simulink model "Interstellar21"  (R2020a)
settings: Solver=ode3  StartTime=0  StopTime=TFinal  FixedStep=Ts  RelTol=1e-3  EnableMultiTasking=on
undefined symbols (not defined in the file or in its folder): bbox_edge_distance_threshold, g, gray, max_num_blobs, Rec, rho, SDTV, sensorCalibrationData, Sensors, sigbuilder_block, States, strel, takeOffDuration
libraries: simulink x14, liblinearframe x1, libraries_plantLibrary x1, visionfilter x1, visionmorphops x1, visionanalysis x1, visionstatistics x1, visiontextngfix x1, visionconversions x1, sensorsLibrary x1
settings Model: Creator=The MathWorks, Inc.  LastModifiedBy=User
settings DataIOCC: LimitDataPoints=on  SaveFormat=Array  SaveOutput=off  SignalLogging=off  DSMLogging=off  SaveTime=off  ReturnWorkspaceOutputs=off
settings OptimizationCC: BlockReduction=off  BufferReuse=off  LifeSpan=inf
settings DebuggingCC: AlgebraicLoopMsg=none  ParameterPrecisionLossMsg=none  UnconnectedInputMsg=none  UnconnectedOutputMsg=none  UnconnectedLineMsg=none  AllowSymbolicDim=off  SFUnexpectedBacktrackingDiag=warning  SFNoUnconditionalDefaultTransitionDiag=warning  SFExecutionAtInitializationDiag=none  ArithmeticOperatorsInVariantConditions=warning
settings HardwareCC: ProdBitPerPointer=32  ProdBitPerSizeT=32  ProdBitPerPtrDiffT=32  ProdLargestAtomicFloat=None  ProdIntDivRoundTo=Undefined  ProdEndianess=Unspecified  ProdWordSize=32  ProdHWDeviceType=32-bit Generic
settings ModelReferenceCC: PropagateSignalLabelsOutOfModel=off
settings SFSimCC: SimUseLocalCustomCode=off  CustomCodeUndefinedFunction=UseInterfaceOnly
settings RTWCC: RTWUseLocalCustomCode=off
settings CodeAppCC: StateflowObjectComments=on
settings GRTTargetCC: TargetLangStandard=C89/C90 (ANSI)
settings ConfigComp: CovMetricSettings=dw  CovHtmlReporting=on  CovSaveCumulativeToWorkspaceVar=on  CovSaveSingleToWorkspaceVar=on  CovExternalEMLEnable=off  CovSFcnEnable=off

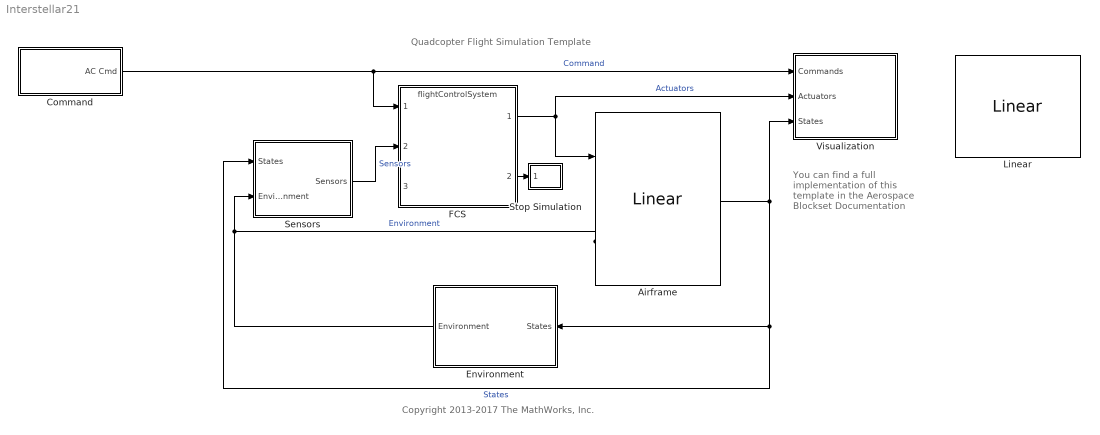
== system Interstellar21 ==
  note: You can find a full implementation of this template in the
      | Aerospace Blockset Documentation
  note: Quadcopter Flight Simulation Template
  note: Copyright 2013-2017 The MathWorks, Inc.
  Airframe : liblinearframe/Linear  SystemSampleTime=-1  Latency=0  AutoFrameSizeCalculation=off
  Command : Subsystem  VariantControl=VSS_COMMAND_SIGBLDR
  Environment : Subsystem  TreatAsAtomicUnit=on  VariantControl=VSS_ENVIRONMENT_CST
  FCS : ModelReference  ModelNameDialog=flightControlSystem.slx  SimulationMode=Normal  ModelReferenceVersion=1.137
  Linear : libraries_plantLibrary/Linear  SystemSampleTime=-1  Latency=0  AutoFrameSizeCalculation=off
  Sensors : Subsystem  TreatAsAtomicUnit=on  VariantControl=VSS_SENSORS_FEEDTHROUGH
  Stop Simulation : Subsystem
  Visualization : Subsystem  VariantControl=VSS_VISUALIZATION_SCOPES
  wires:
  Command/1(AC Cmd) -> Visualization/1(Commands), FCS/1  "Command"
  Sensors/1(Sensors) -> FCS/2  "Sensors"
  FCS/1 -> Airframe/1, Visualization/2(Actuators)  "Actuators"
  Environment/1(Environment) -> Airframe/2, Sensors/2(Environment)  "Environment"
  Airframe/1 -> Visualization/3(States), Environment/1(States), Sensors/1(States)  "States"
  FCS/2 -> Stop Simulation/1(Flag)

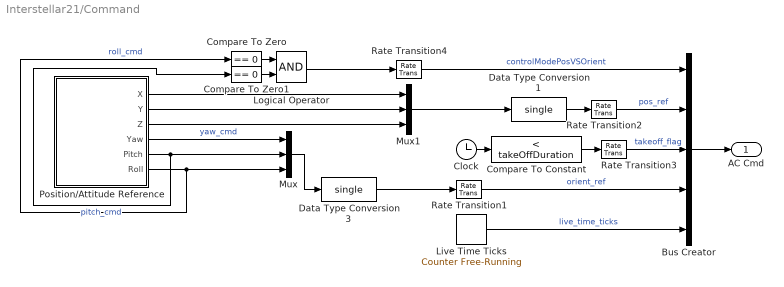
== system Interstellar21/Command ==
  Bus Creator : BusCreator  Inputs=5  OutDataTypeStr=Bus: CommandBus  NonVirtualBus=on
  Clock : Clock
  Compare To Constant : simulink/Logic and Bit Operations/Compare To Constant  relop=<  const=takeOffDuration  OutDataTypeStr=boolean
  Compare To Zero : simulink/Logic and Bit Operations/Compare To Zero  relop===  OutDataTypeStr=boolean
  Compare To Zero1 : simulink/Logic and Bit Operations/Compare To Zero  relop===  OutDataTypeStr=boolean
  Data Type Conversion1 : DataTypeConversion  OutDataTypeStr=single
  Data Type Conversion3 : DataTypeConversion  OutDataTypeStr=single
  Live Time Ticks : simulink/Sources/Counter Free-Running  NumBits=32  tsamp=Ts
  Logical Operator : Logic  AllPortsSameDT=off  OutDataTypeStr=boolean
  Mux : Mux  Inputs=3
  Mux1 : Mux  Inputs=3
  Position/Attitude Reference : Subsystem  Tag=STV Subsys  LoadFcn=sigbuilder_block('load');  StartFcn=sigbuilder_block('start');  StopFcn=sigbuilder_block('stop');  ClipboardFcn=sigbuilder_block('clipboard');  mask(Sigbuilder block){tuvar=[0:10]}
      mask help: Simulink:masks:SigbuilderBlock_MD
      mask init:
      | if ~strcmp(get_param(bdroot(gcbh),'SimulationStatus'),'stopped') tuvar = sigbuilder_block('maskInit'); end
      settings: CopyFcn=sigbuilder_block('copy');  DeleteFcn=sigbuilder_block('delete');  ModelCloseFcn=sigbuilder_block('modelClose');  PreSaveFcn=sigbuilder_block('preSave');  PauseFcn=sigbuilder_block('pause');  ContinueFcn=sigbuilder_block('continue');  NameChangeFcn=sigbuilder_block('namechange');  OpenFcn=sigbuilder_block('open',[246 211.5 555 408.75 ]);  CloseFcn=sigbuilder_block('close');
      mask Display: plot(0, 0, 100, 100,[2, 2, 32, 32, 2], [68, 8, 8, 68, 68],[32, 2], [38, 38], [32, 19, 2],[53, 60, 44], [32, 17, 17, 2],[16, 16, 31, 31]);txt = getActiveGroup(gcbh);text(2, 100, txt,'verticalAlignment', 'top');
  Rate Transition{1..4} (4 alike) : RateTransition  OutPortSampleTime=Ts
  AC Cmd : Outport  OutDataTypeStr=Bus: CommandBus  VectorParamsAs1DForOutWhenUnconnected=off
  wires:
  Bus Creator/1 -> AC Cmd/1
  Position/Attitude Reference/6(Roll) -> Compare To Zero/1, Mux/3  "roll_cmd"
  Position/Attitude Reference/5(Pitch) -> Mux/2, Compare To Zero1/1  "pitch_cmd"
  Position/Attitude Reference/4(Yaw) -> Mux/1  "yaw_cmd"
  Mux/1 -> Data Type Conversion3/1
  Data Type Conversion3/1 -> Rate Transition1/1
  Rate Transition1/1 -> Bus Creator/4  "orient_ref"
  Compare To Zero/1 -> Logical Operator/1
  Compare To Zero1/1 -> Logical Operator/2
  Logical Operator/1 -> Rate Transition4/1
  Rate Transition4/1 -> Bus Creator/1  "controlModePosVSOrient"
  Position/Attitude Reference/1(X) -> Mux1/1
  Position/Attitude Reference/2(Y) -> Mux1/2
  Position/Attitude Reference/3(Z) -> Mux1/3
  Mux1/1 -> Data Type Conversion1/1
  Data Type Conversion1/1 -> Rate Transition2/1
  Rate Transition2/1 -> Bus Creator/2  "pos_ref"
  Clock/1 -> Compare To Constant/1
  Compare To Constant/1 -> Rate Transition3/1
  Rate Transition3/1 -> Bus Creator/3  "takeoff_flag"
  Live Time Ticks/1 -> Bus Creator/5  "live_time_ticks"

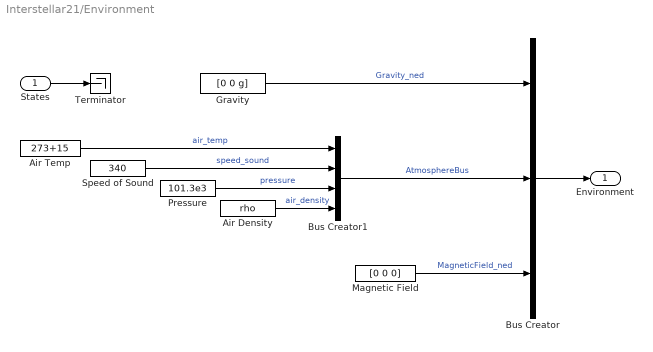
== system Interstellar21/Environment ==
  States : Inport  OutDataTypeStr=Bus: StatesBus
  Air Density : Constant  Value=rho
  Air Temp : Constant  Value=273+15
  Bus Creator : BusCreator  Inputs=3  OutDataTypeStr=Bus: EnvironmentBus  NonVirtualBus=on
  Bus Creator1 : BusCreator  Inputs=4  OutDataTypeStr=Bus: AtmosphereBus  NonVirtualBus=on
  Gravity : Constant  Value=[0 0 g]
  Magnetic Field : Constant  Value=[0 0 0]
  Pressure : Constant  Value=101.3e3
  Speed of Sound : Constant  Value=340
  Terminator : Terminator
  Environment : Outport  VectorParamsAs1DForOutWhenUnconnected=off
  wires:
  States/1 -> Terminator/1
  Gravity/1 -> Bus Creator/1  "Gravity_ned"
  Bus Creator/1 -> Environment/1
  Air Temp/1 -> Bus Creator1/1  "air_temp"
  Speed of Sound/1 -> Bus Creator1/2  "speed_sound"
  Pressure/1 -> Bus Creator1/3  "pressure"
  Air Density/1 -> Bus Creator1/4  "air_density"
  Bus Creator1/1 -> Bus Creator/2  "AtmosphereBus"
  Magnetic Field/1 -> Bus Creator/3  "MagneticField_ned"

== system Interstellar21/Sensors ==
  States : Inport  OutDataTypeStr=Bus: StatesBus
  Environment : Inport  Port=2  OutDataTypeStr=Bus: EnvironmentBus
  Bus Creator1 : BusCreator  Inputs=3  OutDataTypeStr=Bus: SensorsBus  NonVirtualBus=on
  Bus Creator2 : BusCreator  Inputs=3  OutDataTypeStr=Bus: extraSensorData_t  NonVirtualBus=on
  Constant1 : Constant  Value=sensorCalibrationData  OutDataTypeStr=single
  Memory : Memory  InitialCondition=States  InheritSampleTime=on
  Sensor System : Subsystem
  _DUMMY_FLAG_usePosVIS : Constant  Value=Sensors.dummy.usePosVISFlag  OutDataTypeStr=single
  _DUMMY_posVIS : Constant  Value=Sensors.dummy.posVISNoVisionAvail  OutDataTypeStr=single
  Sensors : Outport  OutDataTypeStr=Bus: SensorsBus  VectorParamsAs1DForOutWhenUnconnected=off
  wires:
  Constant1/1 -> Bus Creator1/3  "SensorCalibration"
  Memory/1 -> Sensor System/1(States)
  Sensor System/2(sensordata_data) -> Bus Creator1/2  "HALSensor"
  States/1 -> Memory/1
  Environment/1 -> Sensor System/2(Environment)
  Bus Creator1/1 -> Sensors/1
  _DUMMY_FLAG_usePosVIS/1 -> Bus Creator2/3  "usePosVIS_flag"
  Sensor System/1(opticalFlow_data) -> Bus Creator2/1  "opticalFlow_data"
  _DUMMY_posVIS/1 -> Bus Creator2/2  "posVIS_data"
  Bus Creator2/1 -> Bus Creator1/1  "VisionSensors"

== system Interstellar21/Stop Simulation ==
  Flag : Inport
  Assertion : Assertion
  Compare To Zero : simulink/Logic and Bit Operations/Compare To Zero  relop=>  OutDataTypeStr=boolean
  Logical Operator : Logic  Operator=NOT  AllPortsSameDT=off  OutDataTypeStr=boolean
  wires:
  Flag/1 -> Compare To Zero/1
  Compare To Zero/1 -> Logical Operator/1
  Logical Operator/1 -> Assertion/1

== system Interstellar21/Visualization ==
  Commands : Inport  OutDataTypeStr=Bus: CommandBus
  Actuators : Inport  Port=2
  States : Inport  Port=3  OutDataTypeStr=Bus: StatesBus
  Bus Creator : BusCreator  Inputs=2
  Bus Selector : BusSelector  OutputSignals=States.V_body,States.Euler,States.X_ned
  Euler : Scope
  Motors : Scope
  V_body : Scope
  X_ned : Scope
  wires:
  Commands/1 -> Bus Creator/1  "Commands"
  States/1 -> Bus Creator/2  "States"
  Bus Creator/1 -> Bus Selector/1
  Bus Selector/1 -> V_body/1  "<V_body>"
  Bus Selector/2 -> Euler/1  "<Euler>"
  Bus Selector/3 -> X_ned/1  "<X_ned>"
  Actuators/1 -> Motors/1

== system Interstellar21/Command/Position//Attitude Reference ==
  Demux : Demux  Tag=STV Demux  Outputs=6
      settings: DisplayOption=none
  FromWs : FromWorkspace  Tag=STV FromWs  VariableName=tuvar
      SigBuilderData=|
      | common.afterFinalStr = 'Extrapolate'
      | common.sampleTime = 0
      | dataSet.timeRange = [0 100]
      | dataSet.name = 'Group 1'
      | sbobj.Groups.Name = 'Group 1'
      | sbobj.Groups.Signals(1).Name = 'X'
      | sbobj.Groups.Signals(1).XData = [0 100]
      | sbobj.Groups.Signals(1).YData = [0 0]
      | sbobj.Groups.Signals(2).Name = 'Y'
      | sbobj.Groups.Signals(2).XData = [0 100]
      | sbobj.Groups.Signals(2).YData = [0 0]
      | sbobj.Groups.Signals(3).Name = 'Z'
      | sbobj.Groups.Signals(3).XData = [0 1 1 100]
      | sbobj.Groups.Signals(3).YData = [0 0 -1.5 -1.5]
      | sbobj.Groups.Signals(4).Name = 'Yaw'
      | sbobj.Groups.Signals(4).XData = [0 5.5 8 100]
      | sbobj.Groups.Signals(4).YData = [0 0 0 0]
      | sbobj.Groups.Signals(5).Name = 'Pitch'
      | sbobj.Groups.Signals(5).XData = [0 3 4 100]
      | sbobj.Groups.Signals(5).YData = [0 0 0 0]
      | sbobj.Groups.Signals(6).Name = 'Roll'
      | sbobj.Groups.Signals(6).XData = [0 100]
      | sbobj.Groups.Signals(6).YData = [0 0]
      | sbobj.Groups.TimeRange = [0 100]
  X : Outport  Tag=STV Outport  VectorParamsAs1DForOutWhenUnconnected=off
  Y : Outport  Tag=STV Outport  Port=2  VectorParamsAs1DForOutWhenUnconnected=off
  Z : Outport  Tag=STV Outport  Port=3  VectorParamsAs1DForOutWhenUnconnected=off
  Yaw : Outport  Tag=STV Outport  Port=4  VectorParamsAs1DForOutWhenUnconnected=off
  Pitch : Outport  Tag=STV Outport  Port=5  VectorParamsAs1DForOutWhenUnconnected=off
  Roll : Outport  Tag=STV Outport  Port=6  VectorParamsAs1DForOutWhenUnconnected=off
  wires:
  FromWs/1 -> Demux/1
  Demux/1 -> X/1
  Demux/2 -> Y/1
  Demux/3 -> Z/1
  Demux/4 -> Yaw/1
  Demux/5 -> Pitch/1
  Demux/6 -> Roll/1

== system Interstellar21/Sensors/Sensor System ==
  States : Inport
  Environment : Inport  Port=2
  Camera : Subsystem  AncestorBlock=sensorsLibrary/Camera
  IMU_Pressure : Subsystem
  Rate Transition1 : RateTransition  OutPortSampleTime=Ts
  Rate Transition2 : RateTransition  OutPortSampleTime=Ts
  opticalFlow_data : Outport  VectorParamsAs1DForOutWhenUnconnected=off
  sensordata_data : Outport  Port=2  OutDataTypeStr=Bus: HAL_acquisition_t  VectorParamsAs1DForOutWhenUnconnected=off
  wires:
  Environment/1 -> IMU_Pressure/2(Environment)
  Camera/1(opticalFlow_datout) -> Rate Transition1/1
  IMU_Pressure/1(sensordata_datout) -> Rate Transition2/1
  Rate Transition1/1 -> opticalFlow_data/1
  Rate Transition2/1 -> sensordata_data/1
  States/1 -> Camera/1(states), IMU_Pressure/1(states_datin)

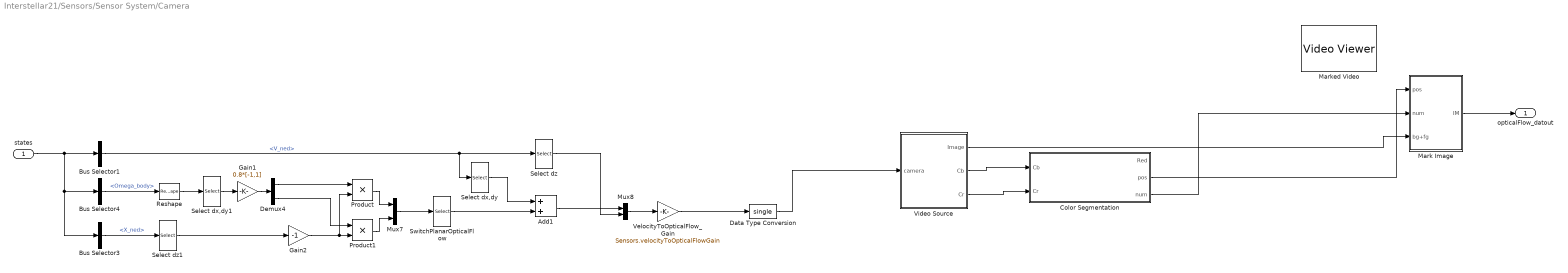
== system Interstellar21/Sensors/Sensor System/Camera ==
  states : Inport
  Add1 : Sum
  Bus Selector1 : BusSelector  OutputSignals=V_ned
  Bus Selector3 : BusSelector  OutputSignals=X_ned
  Bus Selector4 : BusSelector  OutputSignals=Omega_body
  Color Segmentation : Subsystem
  Data Type Conversion : DataTypeConversion  OutDataTypeStr=single
  Demux4 : Demux  Outputs=2
  Gain1 : Gain  Gain=0.8*[-1,1]
  Gain2 : Gain  Gain=-1
  Mark Image : Subsystem
  Marked Video : VideoViewer  colormapValue=gray(256)  FigPos=[410 344 166 142]  trueSizedOnce=on
  Mux7 : Mux  Inputs=2
  Mux8 : Mux  Inputs=2
  Product : Product
  Product1 : Product
  Reshape : Reshape
  Select dx,dy : Selector  InputPortWidth=3  IndexOptions=Index vector (dialog)  Indices=[1 2]  OutputSizes=1
  Select dx,dy1 : Selector  InputPortWidth=3  IndexOptions=Index vector (dialog)  Indices=[1 2]  OutputSizes=1
  Select dz : Selector  InputPortWidth=3  IndexOptions=Index vector (dialog)  Indices=3  OutputSizes=1
  Select dz1 : Selector  InputPortWidth=3  IndexOptions=Index vector (dialog)  Indices=3  OutputSizes=1
  SwitchPlanarOpticalFlow : Selector  InputPortWidth=2  IndexOptions=Index vector (dialog)  Indices=[2 1]  OutputSizes=1
  VelocityToOpticalFlow_Gain : Gain  Gain=Sensors.velocityToOpticalFlowGain
  "Video Source " : Subsystem
  opticalFlow_datout : Outport  VectorParamsAs1DForOutWhenUnconnected=off
  wires:
  Data Type Conversion/1 -> "Video Source "/1("camera ")
  Reshape/1 -> Select dx,dy1/1
  Select dz1/1 -> Gain2/1
  VelocityToOpticalFlow_Gain/1 -> Data Type Conversion/1
  Mux8/1 -> VelocityToOpticalFlow_Gain/1
  Bus Selector4/1 -> Reshape/1  "<Omega_body>"
  Bus Selector3/1 -> Select dz1/1  "<X_ned>"
  Select dz/1 -> Mux8/2
  Add1/1 -> Mux8/1
  SwitchPlanarOpticalFlow/1 -> Add1/2
  Select dx,dy/1 -> Add1/1
  Gain2/1 -> Product1/2, Product/2
  Select dx,dy1/1 -> Gain1/1
  Mux7/1 -> SwitchPlanarOpticalFlow/1
  Product1/1 -> Mux7/2
  Product/1 -> Mux7/1
  Demux4/2 -> Product1/1
  Gain1/1 -> Demux4/1
  Demux4/1 -> Product/1
  Bus Selector1/1 -> Select dz/1, Select dx,dy/1  "<V_ned>"
  states/1 -> Bus Selector1/1, Bus Selector4/1, Bus Selector3/1
  "Video Source "/1(Image) -> Mark Image/3(bg+fg)
  Color Segmentation/2(pos) -> Mark Image/1(pos)
  "Video Source "/3(Cr) -> Color Segmentation/2(Cr)
  Color Segmentation/3(num) -> Mark Image/2(num)
  "Video Source "/2(Cb) -> Color Segmentation/1(Cb)
  Mark Image/1(IM) -> opticalFlow_datout/1

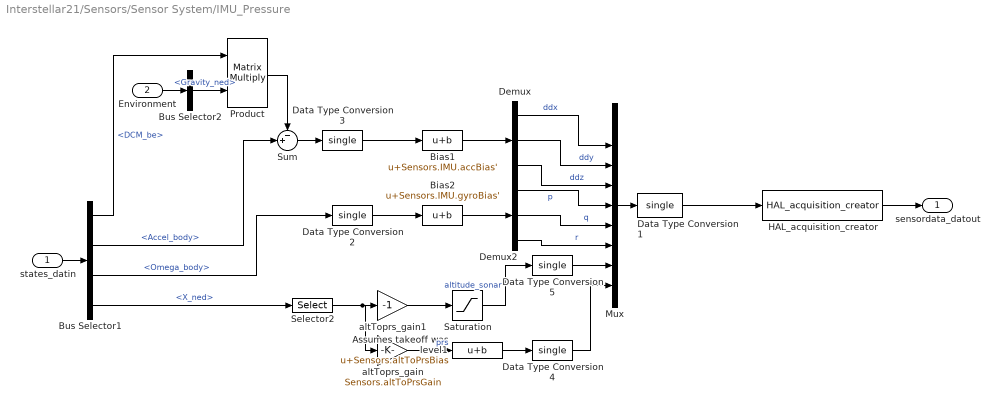
== system Interstellar21/Sensors/Sensor System/IMU_Pressure ==
  states_datin : Inport  OutDataTypeStr=Bus: StatesBus
  Environment : Inport  Port=2
  Assumes takeoff was level1 : Bias  Bias=Sensors.altToPrsBias
  Bias1 : Bias  Bias=Sensors.IMU.accBias'
  Bias2 : Bias  Bias=Sensors.IMU.gyroBias'
  Bus Selector1 : BusSelector  OutputSignals=DCM_be,Accel_body,Omega_body,X_ned
  Bus Selector2 : BusSelector  OutputSignals=Gravity_ned
  Data Type Conversion{1..5} (5 alike) : DataTypeConversion  OutDataTypeStr=single
  Demux : Demux  Outputs=3
  Demux2 : Demux  Outputs=3
  HAL_acquisition_creator : sensorsLibrary/HAL_acquisition_creator  SystemSampleTime=-1  Latency=0  AutoFrameSizeCalculation=off
  Mux : Mux  Inputs=9
  Product : Product  Multiplication=Matrix(*)
  Saturation : Saturate  UpperLimit=inf  LowerLimit=Sensors.altSensorMin  OutDataTypeStr=single
  Selector2 : Selector  InputPortWidth=3  IndexOptions=Index vector (dialog)  Indices=[3]  OutputSizes=1
  Sum : Sum  Inputs=-+|
  altToprs_gain : Gain  Gain=Sensors.altToPrsGain  ParamDataTypeStr=single  OutDataTypeStr=single
  altToprs_gain1 : Gain  Gain=-1  ParamDataTypeStr=single  OutDataTypeStr=single
  sensordata_datout : Outport  OutDataTypeStr=Bus: HAL_acquisition_t  VectorParamsAs1DForOutWhenUnconnected=off
  wires:
  Bias2/1 -> Demux2/1
  Bias1/1 -> Demux/1
  Product/1 -> Sum/1
  Bus Selector1/2 -> Sum/2  "<Accel_body>"
  Sum/1 -> Data Type Conversion3/1
  Bus Selector1/1 -> Product/1  "<DCM_be>"
  Bus Selector2/1 -> Product/2  "<Gravity_ned>"
  altToprs_gain1/1 -> Saturation/1
  Data Type Conversion5/1 -> Mux/8
  Data Type Conversion4/1 -> Mux/9
  Data Type Conversion2/1 -> Bias2/1
  Data Type Conversion3/1 -> Bias1/1
  Assumes takeoff was level1/1 -> Data Type Conversion4/1
  Bus Selector1/4 -> Selector2/1  "<X_ned>"
  states_datin/1 -> Bus Selector1/1
  Environment/1 -> Bus Selector2/1
  Bus Selector1/3 -> Data Type Conversion2/1  "<Omega_body>"
  HAL_acquisition_creator/1 -> sensordata_datout/1
  Data Type Conversion1/1 -> HAL_acquisition_creator/1
  Mux/1 -> Data Type Conversion1/1
  altToprs_gain/1 -> Assumes takeoff was level1/1  "prs"
  Saturation/1 -> Data Type Conversion5/1  "altitude_sonar"
  Selector2/1 -> altToprs_gain1/1, altToprs_gain/1
  Demux/3 -> Mux/4  "ddz"
  Demux2/3 -> Mux/7  "r"
  Demux/2 -> Mux/3  "ddy"
  Demux/1 -> Mux/2  "ddx"
  Demux2/1 -> Mux/5  "p"
  Demux2/2 -> Mux/6  "q"

== system Interstellar21/Sensors/Sensor System/Camera/Color Segmentation ==
  Cb : Inport
  Cr : Inport  Port=2
  Color Classifier : Subsystem
  Filtering : Subsystem
  Region Filtering : Subsystem
  "Red " : Outport
  pos : Outport  Port=2
  num : Outport  Port=3
  wires:
  Color Classifier/1("Red ") -> Filtering/1(Red)
  Filtering/1("refined Red ") -> "Red "/1, Region Filtering/1(Red)
  Cb/1 -> Color Classifier/1(cb)
  Cr/1 -> Color Classifier/2(cr)
  Region Filtering/1(Regions) -> pos/1
  Region Filtering/2(Count) -> num/1

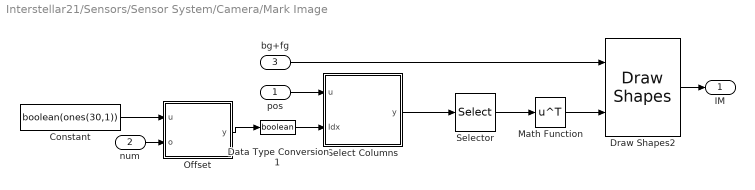
== system Interstellar21/Sensors/Sensor System/Camera/Mark Image ==
  pos : Inport
  num : Inport  Port=2
  bg+fg : Inport  Port=3
  Constant : Constant  Value=boolean(ones(30,1))
  Data Type Conversion1 : DataTypeConversion  OutDataTypeStr=boolean
  Draw Shapes2 : visiontextngfix/Draw Shapes  shape=Lines  fill=off  lineWidth=1  fillClrSource=Specify via dialog  display=User-specified value  intensity=200  color=[0 1 1]  opacity=0.6  viewport=Entire image  antialiasing=off  inType=Obsolete  imagePorts=One multidimensional signal  roundingMode=Floor  overflowMode=off  memoryMode=Specify word length  memoryWordLength=16  prodOutputMode=Binary point scaling  prodOutputWordLength=32  prodOutputFracLength=14  memoryFracLength=15
  Math Function : Math  Operator=transpose  SignedPower=on  SaturateOnIntegerOverflow=on
  Offset : MATLAB Function  TreatAsAtomicUnit=on
  Select Columns : MATLAB Function  TreatAsAtomicUnit=on
  Selector : Selector  NumberOfDimensions=2  InputPortWidth=3  IndexOptions=Index vector (dialog),Select all  Indices=[2 1 4 3],1  OutputSizes=1,1
  IM : Outport
  wires:
  Draw Shapes2/1 -> IM/1
  Data Type Conversion1/1 -> Select Columns/2(Idx)
  Constant/1 -> Offset/1(u)
  pos/1 -> Select Columns/1(u)
  num/1 -> Offset/2(o)
  bg+fg/1 -> Draw Shapes2/1
  Selector/1 -> Math Function/1
  Select Columns/1(y) -> Selector/1
  Math Function/1 -> Draw Shapes2/2
  Offset/1(y) -> Data Type Conversion1/1

== system Interstellar21/Sensors/Sensor System/Camera/Video Source  ==
  "camera " : Inport
  Color Space Conversion : visionconversions/Color Space  Conversion  conversion=Obsolete  conversionActive=R'G'B' to Y'CbCr  wp_str=D65  rec=Rec. 601 (SDTV)  sys=1125/60/2:1  imagePorts=One multidimensional signal
  Select Cb : Selector  NumberOfDimensions=3  InputPortWidth=3  IndexOptions=Select all,Select all,Index vector (dialog)  Indices=[1 3],1,2  OutputSizes=1,1,1
  Select Cr : Selector  NumberOfDimensions=3  InputPortWidth=3  IndexOptions=Select all,Select all,Index vector (dialog)  Indices=[1 3],1,3  OutputSizes=1,1,1
  Image : Outport
  Cb : Outport  Port=2
  Cr : Outport  Port=3
  wires:
  "camera "/1 -> Image/1, Color Space Conversion/1
  Color Space Conversion/1 -> Select Cb/1, Select Cr/1
  Select Cb/1 -> Cb/1
  Select Cr/1 -> Cr/1

== system Interstellar21/Sensors/Sensor System/Camera/Color Segmentation/Color Classifier ==
  cb : Inport
  cr : Inport  Port=2
  2-D FIR Filter : visionfilter/2-D FIR Filter  separable=off  filtSrc=Specify via dialog  filterMtrx=single(1/9*ones(3))  verticalFilter=[4 0]  horizontalFilter=[4 0]  outSize=Full  padType=Constant  padSrc=Specify via dialog  padVal=0  method=Convolution  firstCoeffSignedness=Signed  firstCoeffLastDataTypeStr=Inherit: Same word length as input  outputMode=Binary point scaling  outputWordLength=32  outputFracLength=12  outputSignedness=Auto  outputLastDataTypeStr=fixdt([],32,12)  accumLastDataTypeStr=Inherit: Same as product output  prodOutputMode=Binary point scaling  prodOutputWordLength=32  prodOutputFracLength=10  prodOutputLastDataTypeStr=fixdt([],32,10)  roundingMode=Floor  overflowMode=off  firstCoeffDataTypeStr=Inherit: Same word length as input  firstCoeffMin=[]  firstCoeffMax=[]  prodOutputDataTypeStr=fixdt([],32,10)  accumDataTypeStr=Inherit: Same as product output  outputDataTypeStr=fixdt([],32,12)  outputMin=[]  outputMax=[]
      settings: SourceProductBaseCode=VP
  Compare To Constant1 : simulink/Logic and Bit Operations/Compare To Constant  relop=<  const=2.5  OutDataTypeStr=boolean  ZeroCross=off
  "Mahalanobis Distance " : Subsystem
  "Red " : Outport
  wires:
  "Mahalanobis Distance "/1(Distance) -> 2-D FIR Filter/1
  cb/1 -> "Mahalanobis Distance "/1(Cb)
  cr/1 -> "Mahalanobis Distance "/2(Cr)
  Compare To Constant1/1 -> "Red "/1
  2-D FIR Filter/1 -> Compare To Constant1/1

== system Interstellar21/Sensors/Sensor System/Camera/Color Segmentation/Filtering ==
  Red : Inport
  Closing : visionmorphops/Closing  nhoodsrc=Specify via dialog  strel=strel('disk',5)
      settings: SourceProductBaseCode=VP
  Median Filter : Subsystem
  "refined Red " : Outport
  wires:
  Red/1 -> Median Filter/1(Red)
  Median Filter/1("Filtered Red ") -> Closing/1
  Closing/1 -> "refined Red "/1

== system Interstellar21/Sensors/Sensor System/Camera/Color Segmentation/Region Filtering ==
  Red : Inport
  Blob Analysis : visionstatistics/Blob Analysis  Tag=vipblks_row_conv  area=off  centroid=off  bBox=on  majorAxis=off  minorAxis=off  angle=off  eccentricity=off  equivDiameterSq=off  extent=off  perimeter=off  outDT=single  conn=8  isLabel=off  maxBlobs=max_num_blobs  warnIfNumBlobsExceeded=on  isCount=off  useMinArea=off  minArea=0  useMaxArea=off  maxArea=inf  excludeBorderBlob=off  isOutVarDim=on  isFill=on  fillValues=0  roundingMode=Floor  overflowMode=off  prodOutputMode=Binary point scaling  prodOutputWordLength=32  prodOutputFracLength=16  accumMode=Binary point scaling  accumWordLength=32  accumFracLength=0  outputMode=Binary point scaling  outputWordLength=32  outputFracLength=16  firstCoeffMode=Binary point scaling  firstCoeffWordLength=16  firstCoeffFracLength=14  secondCoeffMode=Binary point scaling  secondCoeffWordLength=32  secondCoeffFracLength=16
  "Extract position " : Subsystem
  Math Function : Math  Operator=transpose  SignedPower=on  SaturateOnIntegerOverflow=on
  Selector : Selector  NumberOfDimensions=2  InputPortWidth=3  IndexOptions=Select all,Index vector (dialog)  Indices=[2 1 4 3],[2 1 4 3]  OutputSizes=1,1
  row3 : Selector  NumberOfDimensions=2  InputPortWidth=3  IndexOptions=Index vector (dialog),Select all  Indices=3,1  OutputSizes=1,1
  row4 : Selector  NumberOfDimensions=2  InputPortWidth=3  IndexOptions=Index vector (dialog),Select all  Indices=4,1  OutputSizes=1,1
  Regions : Outport
  Count : Outport  Port=2
  wires:
  row4/1 -> "Extract position "/2(dc)
  row3/1 -> "Extract position "/1(dr)
  "Extract position "/2(Out2) -> Count/1
  "Extract position "/1(Out1) -> Regions/1
  Red/1 -> Blob Analysis/1
  Selector/1 -> Math Function/1
  Blob Analysis/1 -> Selector/1
  Math Function/1 -> "Extract position "/3(bbox), row4/1, row3/1

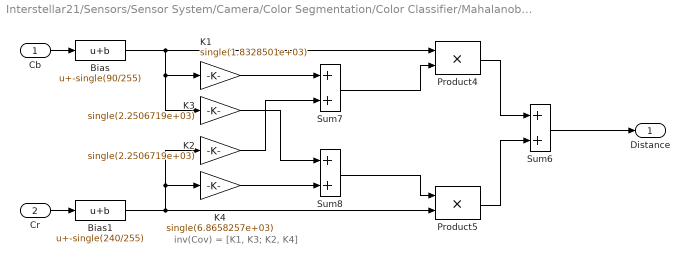
== system Interstellar21/Sensors/Sensor System/Camera/Color Segmentation/Color Classifier/Mahalanobis Distance  ==
  note: inv(Cov) = [K1, K3; K2, K4]
  Cb : Inport
  Cr : Inport  Port=2
  Bias : Bias  Bias=-single(90/255)
  Bias1 : Bias  Bias=-single(240/255)
  K1 : Gain  Gain=single(1.8328501e+03)  SaturateOnIntegerOverflow=on  OutDataTypeStr=Inherit: Same as input  ParamDataTypeStr=Inherit: Same as input
  K2 : Gain  Gain=single(2.2506719e+03)  SaturateOnIntegerOverflow=on  OutDataTypeStr=Inherit: Same as input  ParamDataTypeStr=Inherit: Same as input
  K3 : Gain  Gain=single(2.2506719e+03)  SaturateOnIntegerOverflow=on  OutDataTypeStr=Inherit: Same as input  ParamDataTypeStr=Inherit: Same as input
  K4 : Gain  Gain=single(6.8658257e+03)  SaturateOnIntegerOverflow=on  OutDataTypeStr=Inherit: Same as input  ParamDataTypeStr=Inherit: Same as input
  Product4 : Product  InputSameDT=on  SaturateOnIntegerOverflow=on  OutDataTypeStr=Inherit: Same as first input
  Product5 : Product  InputSameDT=on  SaturateOnIntegerOverflow=on  OutDataTypeStr=Inherit: Same as first input
  Sum6 : Sum  InputSameDT=on  SaturateOnIntegerOverflow=on  OutDataTypeStr=Inherit: Same as first input
  Sum7 : Sum  InputSameDT=on  SaturateOnIntegerOverflow=on  OutDataTypeStr=Inherit: Same as first input
  Sum8 : Sum  InputSameDT=on  SaturateOnIntegerOverflow=on  OutDataTypeStr=Inherit: Same as first input
  Distance : Outport
  wires:
  Cb/1 -> Bias/1
  Cr/1 -> Bias1/1
  K4/1 -> Sum8/2
  Product4/1 -> Sum6/1
  Product5/1 -> Sum6/2
  K1/1 -> Sum7/1
  K2/1 -> Sum7/2
  K3/1 -> Sum8/1
  Sum7/1 -> Product4/2
  Sum8/1 -> Product5/1
  Bias/1 -> Product4/1, K1/1, K3/1
  Bias1/1 -> Product5/2, K4/1, K2/1
  Sum6/1 -> Distance/1

== system Interstellar21/Sensors/Sensor System/Camera/Color Segmentation/Filtering/Median Filter ==
  Red : Inport
  Data Type Conversion5 : DataTypeConversion  OutDataTypeStr=boolean  SaturateOnIntegerOverflow=on  RndMeth=Zero
  Data Type Conversion6 : DataTypeConversion  OutDataTypeStr=single  SaturateOnIntegerOverflow=on  RndMeth=Zero
  Median Filter : visionanalysis/Median Filter  nghbood=[3 3]  outSize=Same as input port I  padType=Constant  padSrc=Specify via dialog  padVal=0  roundingMode=Floor  overflowMode=off
      settings: SourceProductBaseCode=VP
  "Filtered Red " : Outport
  wires:
  Red/1 -> Data Type Conversion6/1
  Data Type Conversion5/1 -> "Filtered Red "/1
  Median Filter/1 -> Data Type Conversion5/1
  Data Type Conversion6/1 -> Median Filter/1

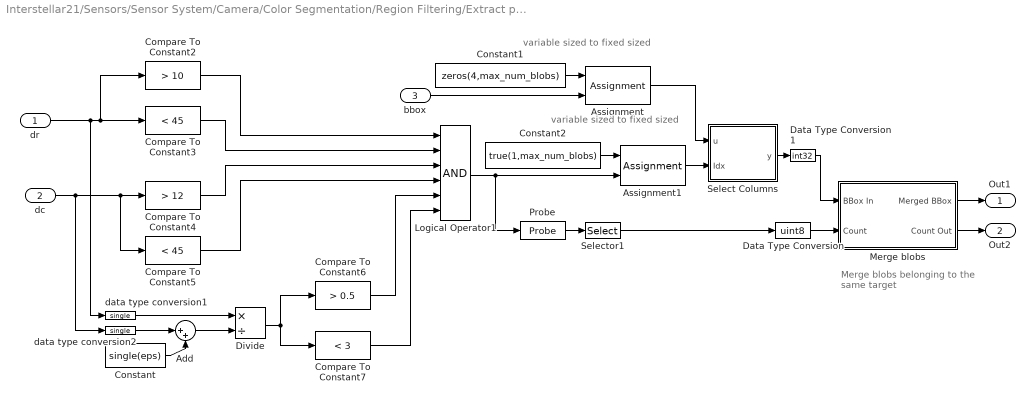
== system Interstellar21/Sensors/Sensor System/Camera/Color Segmentation/Region Filtering/Extract position  ==
  note: Merge blobs belonging
      | to the same target
  note: variable sized to fixed sized
  note: variable sized to fixed sized
  dr : Inport
  dc : Inport  Port=2
  bbox : Inport  Port=3
  Add : Sum  Inputs=|++
  Assignment : Assignment  NumberOfDimensions=2  IndexMode=Zero-based  OutputInitialize=Specify size for each dimension in table  IndexOptions=Assign all,Starting index (dialog)  Indices=0,0  OutputSizes=1,1
  Assignment1 : Assignment  NumberOfDimensions=2  IndexMode=Zero-based  OutputInitialize=Specify size for each dimension in table  IndexOptions=Assign all,Starting index (dialog)  Indices=0,0  OutputSizes=1,1
  Compare To Constant2 : simulink/Logic and Bit Operations/Compare To Constant  relop=>  const=10  OutDataTypeStr=boolean  ZeroCross=off
  Compare To Constant3 : simulink/Logic and Bit Operations/Compare To Constant  relop=<  const=45  OutDataTypeStr=boolean  ZeroCross=off
  Compare To Constant4 : simulink/Logic and Bit Operations/Compare To Constant  relop=>  const=12  OutDataTypeStr=boolean  ZeroCross=off
  Compare To Constant5 : simulink/Logic and Bit Operations/Compare To Constant  relop=<  const=45  OutDataTypeStr=boolean  ZeroCross=off
  Compare To Constant6 : simulink/Logic and Bit Operations/Compare To Constant  relop=>  const=0.5  OutDataTypeStr=boolean  ZeroCross=off
  Compare To Constant7 : simulink/Logic and Bit Operations/Compare To Constant  relop=<  const=3  OutDataTypeStr=boolean  ZeroCross=off
  Constant : Constant  Value=single(eps)
  Constant1 : Constant  Value=zeros(4,max_num_blobs)  OutDataTypeStr=int32
  Constant2 : Constant  Value=true(1,max_num_blobs)  VectorParams1D=off
  Data Type Conversion : DataTypeConversion  OutDataTypeStr=uint8
  Data Type Conversion1 : DataTypeConversion  OutDataTypeStr=int32
  Divide : Product  Inputs=*/
  Logical Operator1 : Logic  Inputs=6  AllPortsSameDT=off  OutDataTypeStr=boolean
  Merge blobs : Subsystem
  Probe : Probe  ProbeWidth=off  ProbeSampleTime=off  ProbeComplexSignal=off  ProbeSignalDimensions=on  ProbeWidthDataType=uint8
  Select Columns : MATLAB Function  TreatAsAtomicUnit=on
  Selector1 : Selector  NumberOfDimensions=2  InputPortWidth=3  IndexOptions=Index vector (dialog),Index vector (dialog)  Indices=1,2  OutputSizes=99,1
  data type conversion1 : DataTypeConversion  OutDataTypeStr=single  SaturateOnIntegerOverflow=on  RndMeth=Zero
  data type conversion2 : DataTypeConversion  OutDataTypeStr=single  SaturateOnIntegerOverflow=on  RndMeth=Zero
  Out1 : Outport
  Out2 : Outport  Port=2
  wires:
  Merge blobs/1(Merged BBox) -> Out1/1
  data type conversion2/1 -> Add/1
  data type conversion1/1 -> Divide/1
  Compare To Constant7/1 -> Logical Operator1/6
  Compare To Constant6/1 -> Logical Operator1/5
  Divide/1 -> Compare To Constant7/1, Compare To Constant6/1
  Add/1 -> Divide/2
  dc/1 -> Compare To Constant4/1, Compare To Constant5/1, data type conversion2/1
  Compare To Constant5/1 -> Logical Operator1/4
  Compare To Constant4/1 -> Logical Operator1/3
  Compare To Constant3/1 -> Logical Operator1/2
  Compare To Constant2/1 -> Logical Operator1/1
  dr/1 -> Compare To Constant2/1, Compare To Constant3/1, data type conversion1/1
  Merge blobs/2(Count Out) -> Out2/1
  Data Type Conversion1/1 -> Merge blobs/1(BBox In)
  Constant/1 -> Add/2
  bbox/1 -> Assignment/2
  Constant1/1 -> Assignment/1
  Constant2/1 -> Assignment1/1
  Logical Operator1/1 -> Assignment1/2, Probe/1
  Assignment/1 -> Select Columns/1(u)
  Assignment1/1 -> Select Columns/2(Idx)
  Probe/1 -> Selector1/1
  Selector1/1 -> Data Type Conversion/1
  Data Type Conversion/1 -> Merge blobs/2(Count)
  Select Columns/1(y) -> Data Type Conversion1/1

== system Interstellar21/Sensors/Sensor System/Camera/Color Segmentation/Region Filtering/Extract position /Merge blobs ==
  note: Thresholds that determine which boxes
      | should be merged
  note: This switch handles
      | the case when Count = 0
  BBox In : Inport
  Count : Inport  Port=2
  Constant1 : Constant  Value=zeros(1,max_num_blobs)  VectorParams1D=off  OutDataTypeStr=Inherit: Inherit via back propagation
  Constant22 : Constant  Value=bbox_edge_distance_threshold  VectorParams1D=off  OutDataTypeStr=Inherit: Inherit via back propagation
  Data Type Conversion : DataTypeConversion  OutDataTypeStr=int32
  Merge blobs : Subsystem
  Select Columns : MATLAB Function  TreatAsAtomicUnit=on
  Sum of Elements : Sum  Inputs=+
  Switch1 : Switch  Criteria=u2 ~= 0  Threshold=1  ZeroCross=off
  Merged BBox : Outport
  Count Out : Outport  Port=2
  wires:
  Constant22/1 -> Merge blobs/3(Thresholds)
  BBox In/1 -> Merge blobs/1(Pos)
  Data Type Conversion/1 -> Merged BBox/1
  Switch1/1 -> Sum of Elements/1, Select Columns/2(Idx)
  Merge blobs/2(Enable_out) -> Switch1/1
  Merge blobs/1(Pos_out) -> Select Columns/1(u)
  Constant1/1 -> Merge blobs/4(Enable), Switch1/3
  Count/1 -> Merge blobs/2(Num), Switch1/2
  Sum of Elements/1 -> Count Out/1
  Select Columns/1(y) -> Data Type Conversion/1

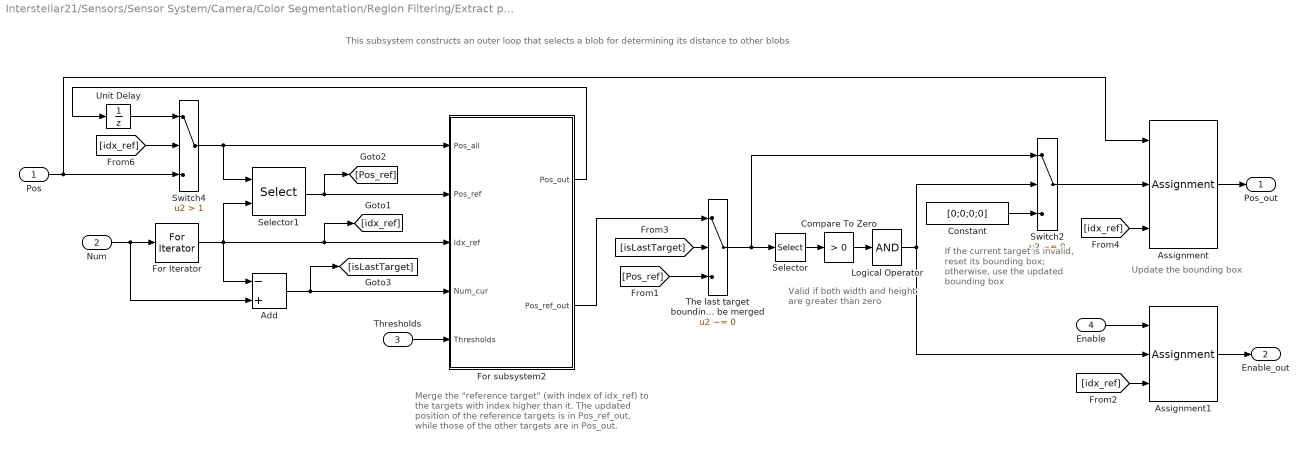
== system Interstellar21/Sensors/Sensor System/Camera/Color Segmentation/Region Filtering/Extract position /Merge blobs/Merge blobs ==
  note: Merge the "reference target" (with index of idx_ref)
      | to the targets with index higher than it.
      | The updated position of the reference targets
      | is in Pos_ref_out, while those of
      | the other targets are in Pos_out.
  note: This subsystem constructs an outer loop that selects a blob for determining its distance to other blobs
  note: Update the bounding box
  note: If the current target is invalid,
      | reset its bounding box;
      | otherwise, use the
      | updated bounding box
  note: Valid if both width and height
      | are greater than zero
  Pos : Inport
  Num : Inport  Port=2
  Thresholds : Inport  Port=3
  Enable : Inport  Port=4
  Add : Sum  Inputs=-+
  Assignment : Assignment  NumberOfDimensions=2  IndexOptions=Assign all,Index vector (port)  Indices=(-1),(-1)  OutputSizes=1, 1
  Assignment1 : Assignment  NumberOfDimensions=2  IndexOptions=Assign all,Index vector (port)  Indices=(-1),(-1)  OutputSizes=1, 1
  Compare To Zero : simulink/Logic and Bit Operations/Compare To Zero  relop=>  OutDataTypeStr=boolean  ZeroCross=off
  Constant : Constant  Value=[0;0;0;0]  OutDataTypeStr=Inherit: Inherit via back propagation
  For Iterator : ForIterator  ResetStates=reset  IterationSource=external
  For subsystem2 : Subsystem
  Logical Operator : Logic  Inputs=1  AllPortsSameDT=off  OutDataTypeStr=boolean
  Selector : Selector  InputPortWidth=4  IndexOptions=Index vector (dialog)  Indices=([3 4])  OutputSizes=1
  Selector1 : Selector  NumberOfDimensions=2  InputPortWidth=3  IndexOptions=Select all,Index vector (port)  Indices=(-1),(-1)  OutputSizes=1
  Switch2 : Switch  Criteria=u2 ~= 0  Threshold=1
  Switch4 : Switch  Criteria=u2 > Threshold  Threshold=1  InputSameDT=on
  The last target bounding box does not need to be merged : Switch  Criteria=u2 ~= 0  Threshold=1
  Unit Delay : UnitDelay  SampleTime=-1  HasFrameUpgradeWarning=on
  Pos_out : Outport
  Enable_out : Outport  Port=2
  wires:
  Enable/1 -> Assignment1/1
  Num/1 -> For Iterator/1, Add/2
  Switch4/1 -> For subsystem2/1(Pos_all), Selector1/1
  Selector1/1 -> For subsystem2/2(Pos_ref), [Pos_ref]
  Assignment1/1 -> Enable_out/1
  Selector/1 -> Compare To Zero/1
  Compare To Zero/1 -> Logical Operator/1
  Thresholds/1 -> For subsystem2/5(Thresholds)
  Unit Delay/1 -> Switch4/1
  Pos/1 -> Switch4/3, Assignment/1
  Logical Operator/1 -> Assignment1/2, Switch2/2
  Constant/1 -> Switch2/3
  Assignment/1 -> Pos_out/1
  [idx_ref] -> Assignment1/3
  For Iterator/1 -> Selector1/2, For subsystem2/3(Idx_ref), [idx_ref], Add/1
  Add/1 -> For subsystem2/4(Num_cur), [isLastTarget]
  [idx_ref] -> Assignment/3
  [idx_ref] -> Switch4/2
  For subsystem2/1(Pos_out) -> Unit Delay/1
  The last target bounding box does not need to be merged/1 -> Switch2/1, Selector/1
  Switch2/1 -> Assignment/2
  For subsystem2/2(Pos_ref_out) -> The last target bounding box does not need to be merged/1
  [isLastTarget] -> The last target bounding box does not need to be merged/2
  [Pos_ref] -> The last target bounding box does not need to be merged/3

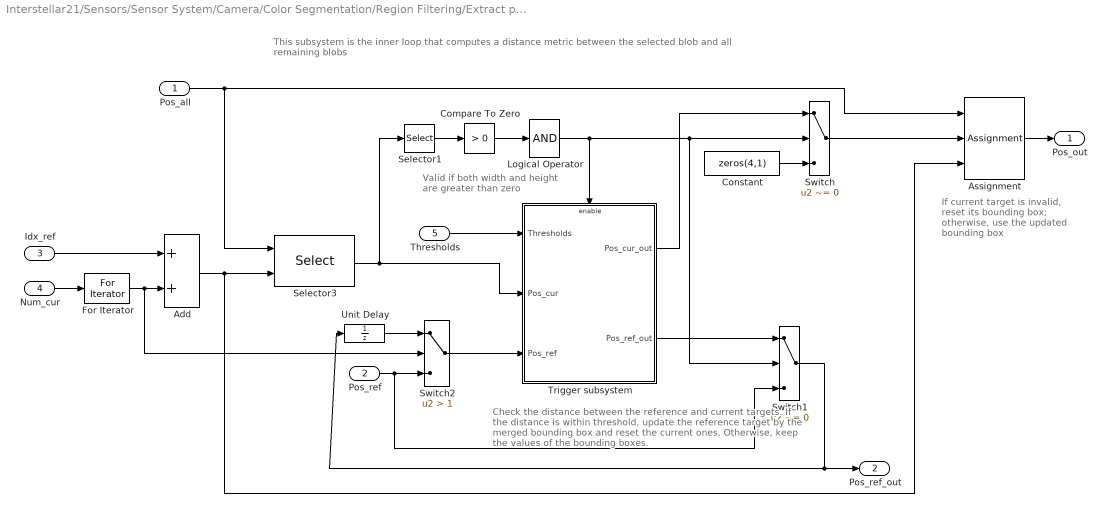
== system Interstellar21/Sensors/Sensor System/Camera/Color Segmentation/Region Filtering/Extract position /Merge blobs/Merge blobs/For subsystem2 ==
  note: Check the distance between the reference and current targets.
      | If the distance is within threshold, update the reference target
      | by the merged bounding box and reset the current ones.
      | Otherwise, keep the values of the bounding boxes.
  note: This subsystem is the inner loop that computes a distance metric between the selected blob and all remaining blobs
  note: If current target is invalid,
      | reset its bounding box;
      | otherwise, use the
      | updated bounding box
  note: Valid if both width and height
      | are greater than zero
  Pos_all : Inport
  Pos_ref : Inport  Port=2
  Idx_ref : Inport  Port=3
  Num_cur : Inport  Port=4
  Thresholds : Inport  Port=5
  Add : Sum
  Assignment : Assignment  NumberOfDimensions=2  IndexOptions=Assign all,Index vector (port)  Indices=(-1),(-1)  OutputSizes=1, 1
  Compare To Zero : simulink/Logic and Bit Operations/Compare To Zero  relop=>  OutDataTypeStr=boolean  ZeroCross=off
  Constant : Constant  Value=zeros(4,1)  VectorParams1D=off  OutDataTypeStr=Inherit: Inherit via back propagation
  For Iterator : ForIterator  ResetStates=reset  IterationSource=external
  Logical Operator : Logic  Inputs=1  AllPortsSameDT=off  OutDataTypeStr=boolean
  Selector1 : Selector  InputPortWidth=4  IndexOptions=Index vector (dialog)  Indices=([3 4])  OutputSizes=1
  Selector3 : Selector  NumberOfDimensions=2  InputPortWidth=3  IndexOptions=Select all,Index vector (port)  Indices=(-1),(-1)  OutputSizes=1
  Switch : Switch  Criteria=u2 ~= 0
  Switch1 : Switch  Criteria=u2 ~= 0
  Switch2 : Switch  Criteria=u2 > Threshold  Threshold=1
  Trigger subsystem : Subsystem
  Unit Delay : UnitDelay  SampleTime=-1  HasFrameUpgradeWarning=on
  Pos_out : Outport
  Pos_ref_out : Outport  Port=2
  wires:
  Pos_ref/1 -> Switch2/3, Switch1/3
  Unit Delay/1 -> Switch2/1
  Constant/1 -> Switch/3
  Trigger subsystem/1(Pos_cur_out) -> Switch/1
  Switch/1 -> Assignment/2
  Switch2/1 -> Trigger subsystem/3(Pos_ref)
  Logical Operator/1 -> Trigger subsystem/Enable, Switch/2, Switch1/2
  Compare To Zero/1 -> Logical Operator/1
  Selector1/1 -> Compare To Zero/1
  Selector3/1 -> Selector1/1, Trigger subsystem/2(Pos_cur)
  Assignment/1 -> Pos_out/1
  Thresholds/1 -> Trigger subsystem/1(Thresholds)
  Add/1 -> Selector3/2, Assignment/3
  Pos_all/1 -> Selector3/1, Assignment/1
  Num_cur/1 -> For Iterator/1
  For Iterator/1 -> Add/2, Switch2/2
  Idx_ref/1 -> Add/1
  Trigger subsystem/2(Pos_ref_out) -> Switch1/1
  Switch1/1 -> Pos_ref_out/1, Unit Delay/1

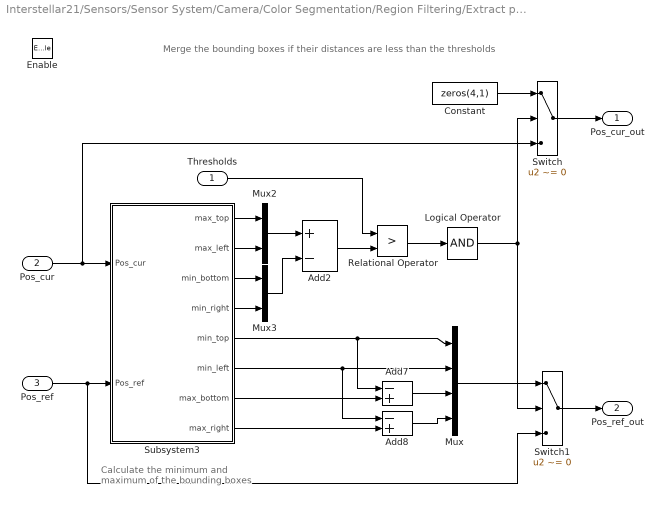
== system Interstellar21/Sensors/Sensor System/Camera/Color Segmentation/Region Filtering/Extract position /Merge blobs/Merge blobs/For subsystem2/Trigger subsystem ==
  note: Calculate the minimum and
      | maximum of the bounding boxes
  note: Merge the bounding boxes if their distances are less than the thresholds
  Thresholds : Inport
  Pos_cur : Inport  Port=2
  Pos_ref : Inport  Port=3
  Enable : EnablePort  PropagateVarSize=During execution
  Add2 : Sum  Inputs=+-
  Add7 : Sum  Inputs=-+
  Add8 : Sum  Inputs=-+
  Constant : Constant  Value=zeros(4,1)  VectorParams1D=off  OutDataTypeStr=Inherit: Inherit via back propagation
  Logical Operator : Logic  Inputs=1  AllPortsSameDT=off  OutDataTypeStr=boolean
  Mux : Mux
  Mux2 : Mux  Inputs=2
  Mux3 : Mux  Inputs=2
  Relational Operator : RelationalOperator  Operator=>  OutDataTypeStr=boolean  RndMeth=Nearest
  Subsystem3 : Subsystem
  Switch : Switch  Criteria=u2 ~= 0
  Switch1 : Switch  Criteria=u2 ~= 0
  Pos_cur_out : Outport
  Pos_ref_out : Outport  Port=2
  wires:
  Add2/1 -> Relational Operator/2
  Mux3/1 -> Add2/2
  Mux2/1 -> Add2/1
  Subsystem3/3(min_bottom) -> Mux3/1
  Subsystem3/4(min_right) -> Mux3/2
  Subsystem3/2(max_left) -> Mux2/2
  Subsystem3/1(max_top) -> Mux2/1
  Logical Operator/1 -> Switch/2, Switch1/2
  Pos_cur/1 -> Switch/3, Subsystem3/1(Pos_cur)
  Switch/1 -> Pos_cur_out/1
  Switch1/1 -> Pos_ref_out/1
  Constant/1 -> Switch/1
  Mux/1 -> Switch1/1
  Add8/1 -> Mux/4
  Add7/1 -> Mux/3
  Subsystem3/8(max_right) -> Add8/2
  Subsystem3/6(min_left) -> Add8/1, Mux/2
  Subsystem3/7(max_bottom) -> Add7/2
  Subsystem3/5(min_top) -> Add7/1, Mux/1
  Pos_ref/1 -> Subsystem3/2(Pos_ref), Switch1/3
  Thresholds/1 -> Relational Operator/1
  Relational Operator/1 -> Logical Operator/1

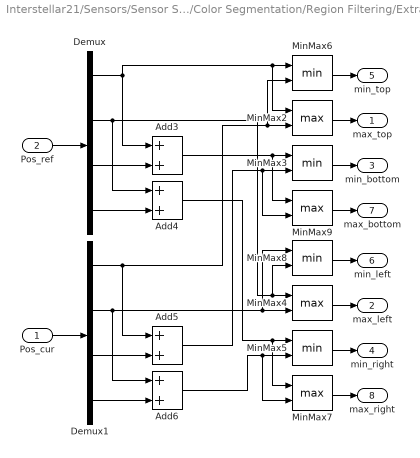
== system Interstellar21/Sensors/Sensor System/Camera/Color Segmentation/Region Filtering/Extract position /Merge blobs/Merge blobs/For subsystem2/Trigger subsystem/Subsystem3 ==
  Pos_cur : Inport
  Pos_ref : Inport  Port=2
  Add{3..6} (4 alike) : Sum
  Demux : Demux
  Demux1 : Demux
  MinMax{2,4,7,9} (4 alike) : MinMax  Function=max  Inputs=2
  MinMax{3,5..6,8} (4 alike) : MinMax  Inputs=2
  max_top : Outport
  max_left : Outport  Port=2
  min_bottom : Outport  Port=3
  min_right : Outport  Port=4
  min_top : Outport  Port=5
  min_left : Outport  Port=6
  max_bottom : Outport  Port=7
  max_right : Outport  Port=8
  wires:
  MinMax7/1 -> max_right/1
  MinMax5/1 -> min_right/1
  MinMax4/1 -> max_left/1
  MinMax8/1 -> min_left/1
  MinMax9/1 -> max_bottom/1
  MinMax3/1 -> min_bottom/1
  MinMax2/1 -> max_top/1
  MinMax6/1 -> min_top/1
  Pos_cur/1 -> Demux1/1
  Pos_ref/1 -> Demux/1
  Demux/2 -> MinMax8/2, MinMax4/1, Add4/1
  Demux/3 -> Add3/2
  Demux/4 -> Add4/2
  Demux1/2 -> MinMax8/1, MinMax4/2, Add6/1
  Demux1/3 -> Add5/2
  Demux1/4 -> Add6/2
  Demux/1 -> MinMax2/1, MinMax6/1, Add3/1
  Demux1/1 -> MinMax6/2, MinMax2/2, Add5/1
  Add3/1 -> MinMax9/1, MinMax3/1
  Add5/1 -> MinMax9/2, MinMax3/2
  Add4/1 -> MinMax7/1, MinMax5/1
  Add6/1 -> MinMax7/2, MinMax5/2

== matlab function Interstellar21/Sensors/Sensor System/Camera/Color Segmentation/Region Filtering/Extract position /Select Columns ==
  data: u input; y output; Idx input
function y = fcn(u, Idx)
%#codegen

y=zeros(size(u));
y(:,1:length(find(Idx))) = u(:,Idx);

== matlab function Interstellar21/Sensors/Sensor System/Camera/Mark Image/Offset ==
  data: u input; y output; o input
function y = fcn(u, o)
%#codegen

y=zeros(size(u));
y(1:o) = u(1:o);

== matlab function Interstellar21/Sensors/Sensor System/Camera/Mark Image/Select Columns ==
  data: u input; y output; Idx input
function y = fcn(u, Idx)
%#codegen

y=zeros(size(u));
y(:,1:length(find(Idx))) = u(:,Idx);

== matlab function Interstellar21/Sensors/Sensor System/Camera/Color Segmentation/Region Filtering/Extract position /Merge blobs/Select Columns ==
  data: u input; y output; Idx input
function y = fcn(u, Idx)
%#codegen

y=zeros(size(u));
y(:,:)=-1;
y(:,1:length(find(Idx))) = u(:,Idx);
